simulink model "compression_chiller_example"  (Simulink 7.6)
settings: Solver=ode45  StartTime=0.0  StopTime=10*3600  RelTol=1e-3
libraries: carnot x3
settings Model: Creator=drhf  LastModifiedBy=drhf

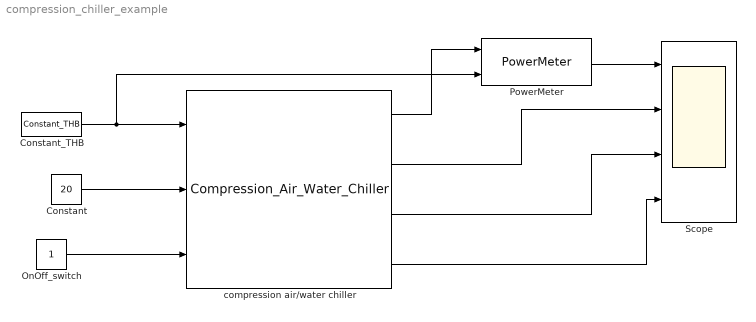
== system compression_chiller_example ==
  Constant : Constant  Value=20
  Constant_THB : carnot/Source/Simple/Constant_THB  SystemSampleTime=-1  t=40  mdot=1000/3600  p=2e5  mID=No Pressure Drop  fluid=water  mix=0  dia=0.02  hgt=0
  OnOff_switch : Constant
      settings: OpenFcn=set_param(gcb,'value',num2str(1-str2num(get_param(gcb,'value'))))
  PowerMeter : carnot/Control/PowerMeter  SystemSampleTime=-1
  Scope : Scope  NumInputPorts=4
      settings: YMin=-5~-5~-5~-5  YMax=5~5~5~5
  compression air/water chiller : carnot/Source/Chiller/Compression_Air_Water_Chiller  SystemSampleTime=-1  Q_Nom=15
  wires:
  Constant_THB/1 -> compression air/water chiller/1, PowerMeter/2
  Constant/1 -> compression air/water chiller/2
  OnOff_switch/1 -> compression air/water chiller/3
  compression air/water chiller/1 -> PowerMeter/1
  PowerMeter/1 -> Scope/1
  compression air/water chiller/2 -> Scope/2
  compression air/water chiller/3 -> Scope/3
  compression air/water chiller/4 -> Scope/4
